simulink model "secondo"  (R2023a)
settings: Solver=VariableStepAuto  StartTime=0.0  StopTime=10  MaxStep=1/1000  RelTol=1e-3
model workspace (MAT data in the model file):
  R0 = 0.05
  R1 = 1
  R2 = 2
  X1 = 2
  X2 = 1
  X3 = 4
  XC = -2
  XM = 1
  n = 2
  w = 6.28318530718
libraries: fl_lib x16, nesl_utility x5
settings Model: Creator=Aguer  LastModifiedBy=Aguer

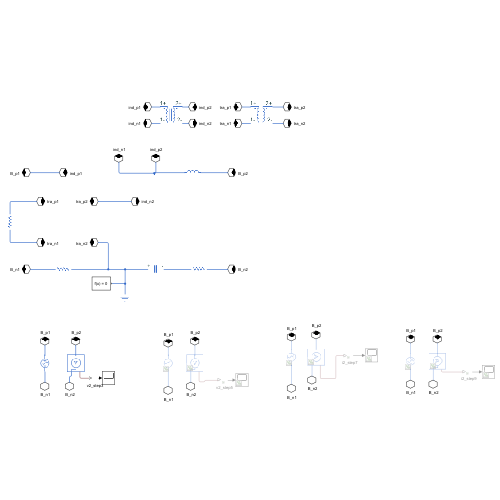
[thumbnail: Simulink's stored preview of the top-level diagram]
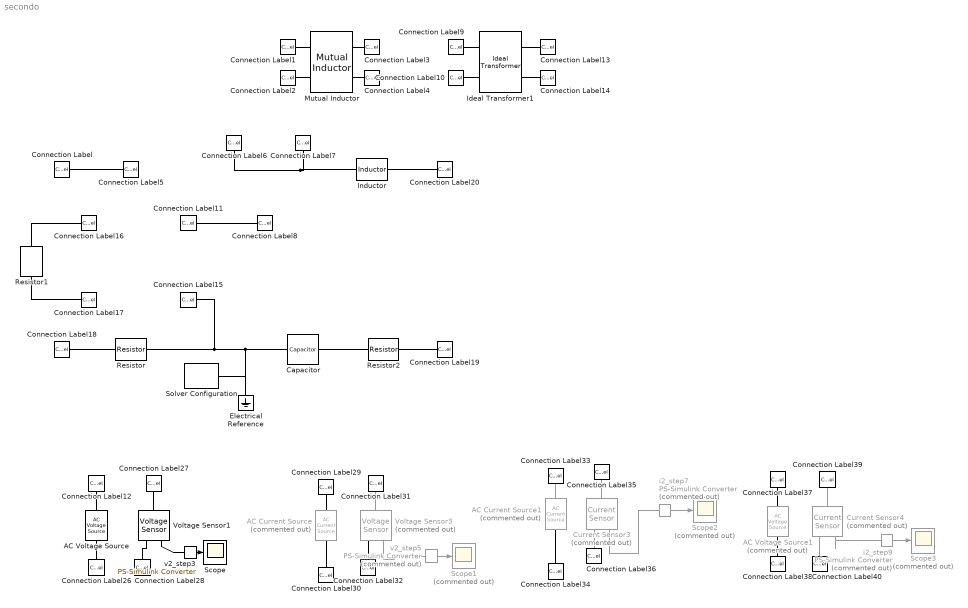
== system secondo ==
  AC Current Source : fl_lib/Electrical/Electrical Sources/AC Current Source  Commented=on  amp=1 A  shift=90 deg  frequency=w/(2*pi) Hz  omega=0 rad/s
      settings: InternalSimscapePortConfiguration="{\"Bottom\":[],\"Left\":[{\"id\":\"p\",\"label\":\"\",\"type\":\"foundation.electrical.electrical\"}],\"Right\":[{\"id\":\"n\",\"label\":\"\",\"type\":\"foundation.electrical.electrical\"}],\"Top\":[]}"
  AC Current Source1 : fl_lib/Electrical/Electrical Sources/AC Current Source  Commented=on  amp=1 A  shift=90 deg  frequency=w/(2*pi) Hz  omega=0 rad/s
      settings: InternalSimscapePortConfiguration="{\"Bottom\":[],\"Left\":[{\"id\":\"p\",\"label\":\"\",\"type\":\"foundation.electrical.electrical\"}],\"Right\":[{\"id\":\"n\",\"label\":\"\",\"type\":\"foundation.electrical.electrical\"}],\"Top\":[]}"
  AC Voltage Source : fl_lib/Electrical/Electrical Sources/AC Voltage Source  amp=1 V  shift=90 deg  frequency=w/(2*pi) Hz  omega=0 rad/s
  AC Voltage Source1 : fl_lib/Electrical/Electrical Sources/AC Voltage Source  Commented=on  amp=1 V  shift=90 deg  frequency=w/(2*pi) Hz  omega=0 rad/s
  Capacitor : fl_lib/Electrical/Electrical Elements/Capacitor  c=-1/(w*XC) F  r=0 Ohm  g=0 1/Ohm  i_specify=off  i_priority=None  i=0 A  i_nominal_specify=off  i_nominal_unit=A  i_nominal_value=1  v_specify=off  v_priority=None  v=0 V  v_nominal_specify=off  v_nominal_unit=V  v_nominal_value=1  vc_specify=off  vc_priority=High  vc=0 V  vc_nominal_specify=off  vc_nominal_unit=V  vc_nominal_value=1
  Connection Label{,12,29,33,37} (5 alike) : ConnectionLabel  Label=B_p1
  Connection Label1 : ConnectionLabel  Label=ind_p1
  Connection Label10 : ConnectionLabel  Label=tra_n1
  Connection Label11 : ConnectionLabel  Label=tra_p2
  Connection Label13 : ConnectionLabel  Label=tra_p2
  Connection Label14 : ConnectionLabel  Label=tra_n2
  Connection Label15 : ConnectionLabel  Label=tra_n2
  Connection Label16 : ConnectionLabel  Label=tra_p1
  Connection Label17 : ConnectionLabel  Label=tra_n1
  Connection Label{18,26,30,34,38} (5 alike) : ConnectionLabel  Label=B_n1
  Connection Label{19,28,32,36,40} (5 alike) : ConnectionLabel  Label=B_n2
  Connection Label2 : ConnectionLabel  Label=ind_n1
  Connection Label{20,27,31,35,39} (5 alike) : ConnectionLabel  Label=B_p2
  Connection Label3 : ConnectionLabel  Label=ind_p2
  Connection Label4 : ConnectionLabel  Label=ind_n2
  Connection Label5 : ConnectionLabel  Label=ind_p1
  Connection Label6 : ConnectionLabel  Label=ind_n1
  Connection Label7 : ConnectionLabel  Label=ind_p2
  Connection Label8 : ConnectionLabel  Label=ind_n2
  Connection Label9 : ConnectionLabel  Label=tra_p1
  Current Sensor3 : fl_lib/Electrical/Electrical Sensors/Current Sensor  Commented=on
  Current Sensor4 : fl_lib/Electrical/Electrical Sensors/Current Sensor  Commented=on
  Electrical Reference : fl_lib/Electrical/Electrical Elements/Electrical Reference
  Ideal Transformer1 : fl_lib/Electrical/Electrical Elements/Ideal Transformer  n=n  i1_specify=off  i1_priority=None  i1=0 A  i1_nominal_specify=off  i1_nominal_unit=A  i1_nominal_value=1  v1_specify=off  v1_priority=None  v1=0 V  v1_nominal_specify=off  v1_nominal_unit=V  v1_nominal_value=1  i2_specify=off  i2_priority=None  i2=0 A  i2_nominal_specify=off  i2_nominal_unit=A  i2_nominal_value=1  v2_specify=off  v2_priority=None  v2=0 V  v2_nominal_specify=off  v2_nominal_unit=V  v2_nominal_value=1
  Inductor : fl_lib/Electrical/Electrical Elements/Inductor  l=X2/w H  r=0 Ohm  g=0 1/Ohm  i_specify=off  i_priority=None  i=0 A  i_nominal_specify=off  i_nominal_unit=A  i_nominal_value=1  v_specify=off  v_priority=None  v=0 V  v_nominal_specify=off  v_nominal_unit=V  v_nominal_value=1  i_L_specify=off  i_L_priority=High  i_L=0 A  i_L_nominal_specify=off  i_L_nominal_unit=A  i_L_nominal_value=1
  Mutual Inductor : fl_lib/Electrical/Electrical Elements/Mutual Inductor  L1=X1/w H  L2=X3/w H  k=XM/((sqrt(X1))*(sqrt(X3)))  i1_specify=off  i1_priority=High  i1=-2 A  i1_nominal_specify=off  i1_nominal_unit=A  i1_nominal_value=1  i2_specify=off  i2_priority=High  i2=0 A  i2_nominal_specify=off  i2_nominal_unit=A  i2_nominal_value=1  v1_specify=off  v1_priority=None  v1=0 V  v1_nominal_specify=off  v1_nominal_unit=V  v1_nominal_value=1  v2_specify=off  v2_priority=None  v2=0 V  v2_nominal_specify=off  v2_nominal_unit=V  v2_nominal_value=1
      settings: InternalSimscapePortConfiguration="{\"Bottom\":[],\"Left\":[{\"id\":\"p1\",\"label\":\"1+\",\"type\":\"foundation.electrical.electrical\"},{\"id\":\"n1\",\"label\":\"1-\",\"type\":\"foundation.electrical.electrical\"}],\"Right\":[{\"id\":\"p2\",\"label\":\"2+\",\"type\":\"foundation.electrical.electrical\"},{\"id\":\"n2\",\"label\":\"2-\",\"type\":\"foundation.electrical.electrical\"}],\"Top\":[]}"
  Resistor : fl_lib/Electrical/Electrical Elements/Resistor  R=R1 Ohm  i_specify=off  i_priority=None  i=0 A  i_nominal_specify=off  i_nominal_unit=A  i_nominal_value=1  v_specify=off  v_priority=None  v=0 V  v_nominal_specify=off  v_nominal_unit=V  v_nominal_value=1
  Resistor1 : fl_lib/Electrical/Electrical Elements/Resistor  R=R0 Ohm  i_specify=off  i_priority=None  i=0 A  i_nominal_specify=off  i_nominal_unit=A  i_nominal_value=1  v_specify=off  v_priority=None  v=0 V  v_nominal_specify=off  v_nominal_unit=V  v_nominal_value=1
  Resistor2 : fl_lib/Electrical/Electrical Elements/Resistor  R=R2 Ohm  i_specify=off  i_priority=None  i=0 A  i_nominal_specify=off  i_nominal_unit=A  i_nominal_value=1  v_specify=off  v_priority=None  v=0 V  v_nominal_specify=off  v_nominal_unit=V  v_nominal_value=1
  Scope : Scope
  Scope1 : Scope  Commented=on
  Scope2 : Scope  Commented=on
  Scope3 : Scope  Commented=on
  Solver Configuration : nesl_utility/Solver Configuration  PhysicalDomain=network_engine_domain  SubClassName=solver  LeftPortType=input  RightPortType=generic  Tones=[]  Harmonics=[]  SimulateNoise=off  Profile=off  UseLocalSampling=off  EnableSwitchedLinearOptims=on  FrequencyDomain=off  UseCCode=off  RelTol=0.001  AbsTol=0.001  MinStep=1e-09  ToWorkspace=off  RevertToSquareIcSolve=off  NumHomotopyIterations=100  PhasorMode=off  PhasorModeNumHarmonics=1  ConsistencySolver=NEWTON_XTOL_AFTER_FTOL  IndexReductionMethod=DerivativeReplacement  DoDC=off  ResidualTolerance=1e-09  ConsistencyTolSource=GLOBAL  ConsistencyAbsTol=0.001  ConsistencyRelTol=0.001  ConsistencyTolFactor=0.001  UseLocalSolver=off  LocalSolverChoice=NE_BACKWARD_EULER_ADVANCER  ResolveIndetEquations=on  FunctionEvalNumThread=1  LocalSolverSampleTime=0.001  DoFixedCost=off  MaxNonlinIter=3  MaxModeIter=2  ComputeImpulses=off  ImpulseIterations=2  LinearAlgebra=auto  LinearAlgebraNumThread=0  EquationFormulation=NE_TIME_EF  DelaysMemoryBudget=1024  AutomaticFiltering=on  FilteringTimeConstant=0.001  PartitionStorageMethod=AS_NEEDED  PartitionMemoryBudget=1024  PartitionMethod=ROBUST
  Voltage Sensor1 : fl_lib/Electrical/Electrical Sensors/Voltage Sensor
  Voltage Sensor3 : fl_lib/Electrical/Electrical Sensors/Voltage Sensor  Commented=on
  i2_step7 : nesl_utility/PS-Simulink Converter  Commented=on  PhysicalDomain=network_engine_domain  SubClassName=ps_output  LeftPortType=input  RightPortType=output  PseudoPeriodic=off  Frequencies=[]  VectorFormat=1-D array  Unit=inherit  AffineConversion=off
  i2_step9 : nesl_utility/PS-Simulink Converter  Commented=on  PhysicalDomain=network_engine_domain  SubClassName=ps_output  LeftPortType=input  RightPortType=output  PseudoPeriodic=off  Frequencies=[]  VectorFormat=1-D array  Unit=inherit  AffineConversion=off
  v2_step3 : nesl_utility/PS-Simulink Converter  PhysicalDomain=network_engine_domain  SubClassName=ps_output  LeftPortType=input  RightPortType=output  PseudoPeriodic=off  Frequencies=[]  VectorFormat=1-D array  Unit=inherit  AffineConversion=off
  v2_step5 : nesl_utility/PS-Simulink Converter  Commented=on  PhysicalDomain=network_engine_domain  SubClassName=ps_output  LeftPortType=input  RightPortType=output  PseudoPeriodic=off  Frequencies=[]  VectorFormat=1-D array  Unit=inherit  AffineConversion=off
  wires:
  v2_step3/1 -> Scope/1
  i2_step9/1 -> Scope3/1
  i2_step7/1 -> Scope2/1
  v2_step5/1 -> Scope1/1
  connections:
  Current Sensor3/LConn1 -- Connection Label35/LConn1
  Current Sensor3/RConn2 -- Connection Label36/LConn1
  Connection Label28/LConn1 -- Voltage Sensor1/RConn2
  Connection Label14/LConn1 -- Ideal Transformer1/RConn2
  Connection Label34/LConn1 -- AC Current Source1/RConn1
  Connection Label9/LConn1 -- Ideal Transformer1/LConn1
  Connection Label37/LConn1 -- AC Voltage Source1/LConn1
  v2_step3/LConn1 -- Voltage Sensor1/RConn1
  Connection Label29/LConn1 -- AC Current Source/LConn1
  Connection Label38/LConn1 -- AC Voltage Source1/RConn1
  v2_step5/LConn1 -- Voltage Sensor3/RConn1
  Current Sensor4/LConn1 -- Connection Label39/LConn1
  Connection Label1/LConn1 -- Mutual Inductor/LConn1
  Connection Label10/LConn1 -- Ideal Transformer1/LConn2
  Connection Label32/LConn1 -- Voltage Sensor3/RConn2
  Connection Label26/LConn1 -- AC Voltage Source/RConn1
  Connection Label3/LConn1 -- Mutual Inductor/RConn1
  Connection Label12/LConn1 -- AC Voltage Source/LConn1
  Ideal Transformer1/RConn1 -- Connection Label13/LConn1
  Current Sensor3/RConn1 -- i2_step7/LConn1
  Current Sensor4/RConn2 -- Connection Label40/LConn1
  Connection Label2/LConn1 -- Mutual Inductor/LConn2
  Voltage Sensor3/LConn1 -- Connection Label31/LConn1
  Voltage Sensor1/LConn1 -- Connection Label27/LConn1
  AC Current Source1/LConn1 -- Connection Label33/LConn1
  Connection Label30/LConn1 -- AC Current Source/RConn1
  Connection Label4/LConn1 -- Mutual Inductor/RConn2
  Current Sensor4/RConn1 -- i2_step9/LConn1
  Connection Label5/LConn1 -- Connection Label/LConn1
  Connection Label7/LConn1 -- Inductor/LConn1 -- Connection Label6/LConn1
  Connection Label15/LConn1 -- Solver Configuration/RConn1 -- Electrical Reference/LConn1 -- Capacitor/LConn1 -- Resistor/RConn1
  Connection Label11/LConn1 -- Connection Label8/LConn1
  Resistor1/LConn1 -- Connection Label16/LConn1
  Resistor1/RConn1 -- Connection Label17/LConn1
  Connection Label18/LConn1 -- Resistor/LConn1
  Resistor2/LConn1 -- Capacitor/RConn1
  Connection Label19/LConn1 -- Resistor2/RConn1
  Connection Label20/LConn1 -- Inductor/RConn1
